simulink model "rigidBodyPD"  (Simulink 6.1)
settings: Solver=ode45  StartTime=0.0  StopTime=20.0  RelTol=1e-3
libraries: simulink x7
settings Model: LastModifiedBy=okawa
settings DebuggingCC: SolverPrmCheckMsg=warning

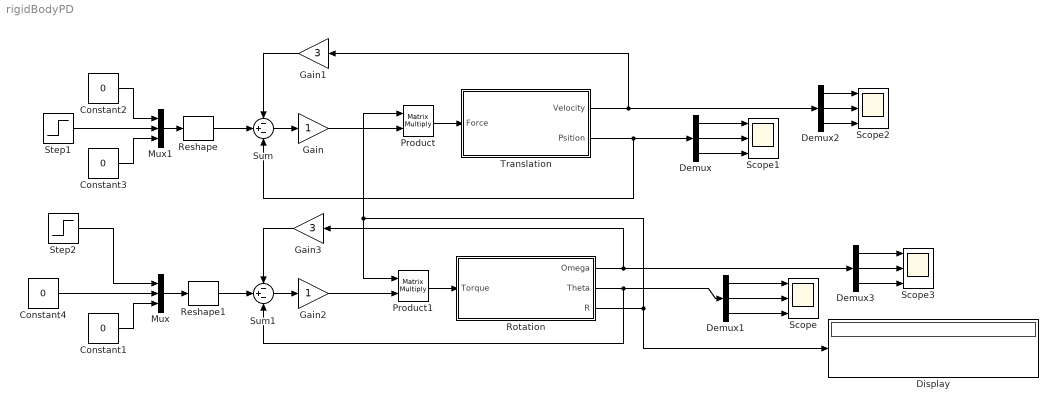
== system rigidBodyPD ==
  Constant{1..4} (4 alike) : Constant  Value=0
  Demux{,1..3} (4 alike) : Demux  Outputs=3
  Display : Display
  Gain : Gain
  Gain1 : Gain  Orientation=left  Gain=3
  Gain2 : Gain
  Gain3 : Gain  Orientation=left  Gain=3
  Mux : Mux  Inputs=3
  Mux1 : Mux  Inputs=3
  Product : Product  Multiplication=Matrix(*)  RndMeth=Zero
  Product1 : Product  Multiplication=Matrix(*)  RndMeth=Zero
  Reshape : simulink/Math Operations/Reshape  OutputDimensionality=Column vector  OutputDimensions=[1,1]
  Reshape1 : simulink/Math Operations/Reshape  OutputDimensionality=Column vector  OutputDimensions=[1,1]
  Rotation : Subsystem
  Scope{,1..3} (4 alike) : Scope  NumInputPorts=3
      Scope settings: YMin=-5~-5~-5  YMax=5~5~5
      Scope1 settings: YMin=-5~-5~-5  YMax=5~5~5
      Scope2 settings: YMin=-5~-5~-5  YMax=5~5~5  SaveName=ScopeData2
      Scope3 settings: YMin=-5~-5~-5  YMax=5~5~5  SaveName=ScopeData3
  Step1 : Step  SampleTime=0
  Step2 : Step  After=0.5  SampleTime=0
  Sum : Sum  Inputs=-+-
  Sum1 : Sum  Inputs=-+-
  Translation : Subsystem
  wires:
  Constant1/1 -> Mux/3
  Constant2/1 -> Mux1/1
  Step1/1 -> Mux1/2
  Constant3/1 -> Mux1/3
  Mux1/1 -> Reshape/1
  Product/1 -> Translation/1(Force)
  Demux1/1 -> Scope/1
  Demux1/2 -> Scope/2
  Demux1/3 -> Scope/3
  Mux/1 -> Reshape1/1
  Product1/1 -> Rotation/1(Torque)
  Translation/2(Psition) -> Demux/1, Sum/3
  Demux2/1 -> Scope2/1
  Demux2/2 -> Scope2/2
  Demux2/3 -> Scope2/3
  Translation/1(Velocity) -> Demux2/1, Gain1/1
  Demux/1 -> Scope1/1
  Demux/2 -> Scope1/2
  Demux/3 -> Scope1/3
  Demux3/1 -> Scope3/1
  Demux3/2 -> Scope3/2
  Demux3/3 -> Scope3/3
  Rotation/1(Omega) -> Demux3/1, Gain3/1
  Rotation/3(R) -> Product/1, Product1/1, Display/1
  Rotation/2(Theta) -> Demux1/1, Sum1/3
  Sum/1 -> Gain/1
  Gain/1 -> Product/2
  Reshape/1 -> Sum/2
  Gain1/1 -> Sum/1
  Reshape1/1 -> Sum1/2
  Sum1/1 -> Gain2/1
  Gain2/1 -> Product1/2
  Gain3/1 -> Sum1/1
  Step2/1 -> Mux/1
  Constant4/1 -> Mux/2

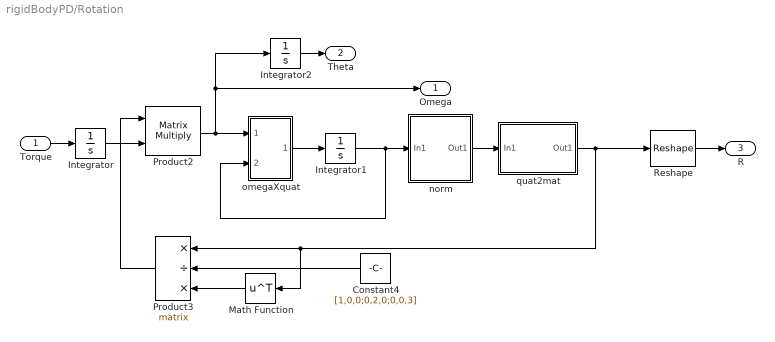
== system rigidBodyPD/Rotation ==
  Torque : Inport  Port=1  LatchInput=off
  Constant4 : Constant  Orientation=left  Value=[1,0,0;0,2,0;0,0,3]  VectorParams1D=off
  Integrator : Integrator
  Integrator1 : Integrator  InitialCondition=[1;0;0;0]
  Integrator2 : Integrator
  Math Function : Math  Orientation=left  Operator=transpose  SaturateOnIntegerOverflow=on
  Product2 : Product  Multiplication=Matrix(*)  RndMeth=Zero
  Product3 : Product  Orientation=left  Inputs=*/*  Multiplication=Matrix(*)  RndMeth=Zero
  Reshape : simulink/Math Operations/Reshape  OutputDimensionality=Customize  OutputDimensions=[3,3]
  norm : Subsystem
  "omegaXquat " : Subsystem
  quat2mat : Subsystem
  Omega : Outport
  Theta : Outport  Port=2
  R : Outport  Port=3
  wires:
  Integrator/1 -> Product2/2
  Product3/1 -> Product2/1
  Product2/1 -> "omegaXquat "/1(In1), Integrator2/1, Omega/1
  "omegaXquat "/1(Out1) -> Integrator1/1
  Integrator1/1 -> "omegaXquat "/2(In2), norm/1(In1)
  quat2mat/1(Out1) -> Product3/1, Math Function/1, Reshape/1
  Constant4/1 -> Product3/2
  Math Function/1 -> Product3/3
  norm/1(Out1) -> quat2mat/1(In1)
  Integrator2/1 -> Theta/1
  Torque/1 -> Integrator/1
  Reshape/1 -> R/1

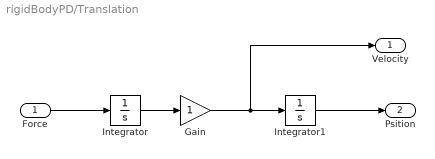
== system rigidBodyPD/Translation ==
  Force : Inport  Port=1  LatchInput=off
  Gain : Gain
  Integrator : Integrator
  Integrator1 : Integrator
  Velocity : Outport
  Psition : Outport  Port=2
  wires:
  Integrator/1 -> Gain/1
  Gain/1 -> Integrator1/1, Velocity/1
  Force/1 -> Integrator/1
  Integrator1/1 -> Psition/1

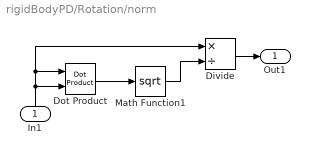
== system rigidBodyPD/Rotation/norm ==
  In1 : Inport  Orientation=up  Port=1  LatchInput=off
  Divide : Product  Inputs=*/  OutScaling=2^-10
  Dot Product : simulink/Math Operations/Dot Product  InputSameDT=on  OutDataType=sfix(16)  OutScaling=2^-10  DoSatur=off
  Math Function1 : Math  Operator=sqrt  SaturateOnIntegerOverflow=on
  Out1 : Outport
  wires:
  Dot Product/1 -> Math Function1/1
  Math Function1/1 -> Divide/2
  In1/1 -> Dot Product/2, Dot Product/1, Divide/1
  Divide/1 -> Out1/1

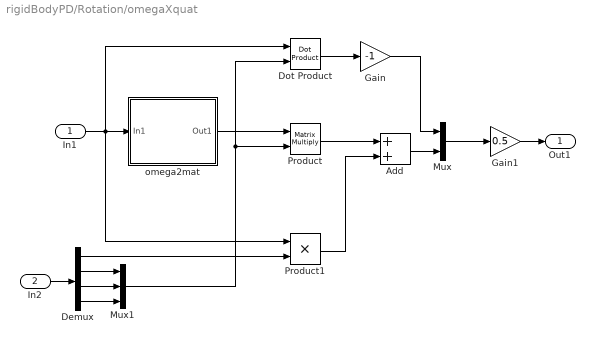
== system rigidBodyPD/Rotation/omegaXquat  ==
  In1 : Inport  Port=1  LatchInput=off
  In2 : Inport  Port=2  LatchInput=off
  Add : Sum  OutScaling=2^-10
  Demux : Demux
  Dot Product : simulink/Math Operations/Dot Product  InputSameDT=on  OutDataType=sfix(16)  OutScaling=2^-10  DoSatur=off
  Gain : Gain  Gain=-1
  Gain1 : Gain  Gain=0.5
  Mux : Mux  Inputs=2
  Mux1 : Mux  Inputs=3
  Product : Product  Multiplication=Matrix(*)  RndMeth=Zero
  Product1 : Product  RndMeth=Zero
  omega2mat : Subsystem
  Out1 : Outport
  wires:
  In1/1 -> Product1/1, Dot Product/1, omega2mat/1(In1)
  Dot Product/1 -> Gain/1
  omega2mat/1(Out1) -> Product/1
  Product/1 -> Add/1
  Product1/1 -> Add/2
  Gain/1 -> Mux/1
  Add/1 -> Mux/2
  Mux/1 -> Gain1/1
  Demux/2 -> Mux1/1
  Demux/3 -> Mux1/2
  Demux/4 -> Mux1/3
  Mux1/1 -> Dot Product/2, Product/2
  Demux/1 -> Product1/2
  Gain1/1 -> Out1/1
  In2/1 -> Demux/1

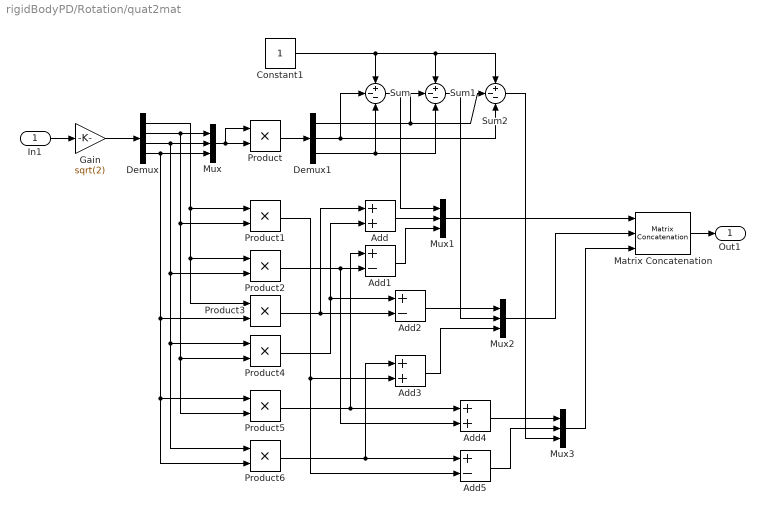
== system rigidBodyPD/Rotation/quat2mat ==
  In1 : Inport  Port=1  LatchInput=off
  Add : Sum  OutScaling=2^-10
  Add1 : Sum  Inputs=+-  OutScaling=2^-10
  Add2 : Sum  Inputs=+-  OutScaling=2^-10
  Add3 : Sum  OutScaling=2^-10
  Add4 : Sum  OutScaling=2^-10
  Add5 : Sum  Inputs=+-  OutScaling=2^-10
  Constant1 : Constant
  Demux : Demux
  Demux1 : Demux  Outputs=3
  Gain : Gain  Gain=sqrt(2)
  Matrix Concatenation : simulink/Math Operations/Matrix Concatenation  numInports=3  catMethod=Horizontal
  Mux{,1..3} (4 alike) : Mux  Inputs=3
  Product{,1..6} (7 alike) : Product  RndMeth=Zero
  Sum : Sum  Inputs=+--
  Sum1 : Sum  Inputs=+--
  Sum2 : Sum  Inputs=+--
  Out1 : Outport
  wires:
  Gain/1 -> Demux/1
  Demux/2 -> Mux/1, Product1/2, Product5/2, Product4/2
  Demux/3 -> Mux/2, Product6/1, Product4/1, Product2/2
  Demux/4 -> Mux/3, Product6/2, Product5/1, Product3/2
  Mux/1 -> Product/2, Product/1
  Product/1 -> Demux1/1
  Constant1/1 -> Sum/1, Sum2/1, Sum1/1
  Demux1/1 -> Sum2/2, Sum1/2
  Demux1/2 -> Sum2/3, Sum/2
  Demux1/3 -> Sum1/3, Sum/3
  Demux/1 -> Product1/1, Product3/1, Product2/1
  Mux1/1 -> Matrix Concatenation/1
  Mux3/1 -> Matrix Concatenation/3
  Mux2/1 -> Matrix Concatenation/2
  Add4/1 -> Mux3/1
  Add5/1 -> Mux3/2
  Sum2/1 -> Mux3/3
  Product6/1 -> Add5/1, Add3/1
  Product1/1 -> Add5/2, Add3/2
  Product5/1 -> Add4/1, Add1/1
  Add2/1 -> Mux2/1
  Sum1/1 -> Mux2/2
  Add3/1 -> Mux2/3
  Sum/1 -> Mux1/1
  Add/1 -> Mux1/2
  Add1/1 -> Mux1/3
  Product3/1 -> Add2/2, Add/1
  Product4/1 -> Add/2, Add2/1
  Product2/1 -> Add1/2, Add4/2
  In1/1 -> Gain/1
  Matrix Concatenation/1 -> Out1/1

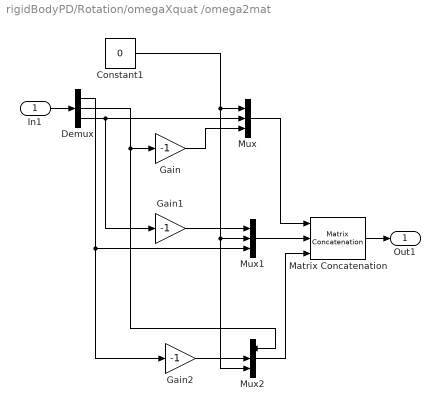
== system rigidBodyPD/Rotation/omegaXquat /omega2mat ==
  In1 : Inport  Port=1  LatchInput=off
  Constant1 : Constant  Value=0
  Demux : Demux  Outputs=3
  Gain : Gain  Gain=-1
  Gain1 : Gain  Gain=-1
  Gain2 : Gain  Gain=-1
  Matrix Concatenation : simulink/Math Operations/Matrix Concatenation  numInports=3  catMethod=Horizontal
  Mux : Mux  Inputs=3
  Mux1 : Mux  Inputs=3
  Mux2 : Mux  Inputs=3
  Out1 : Outport
  wires:
  Constant1/1 -> Mux/1, Mux1/2, Mux2/3
  Demux/2 -> Gain/1, Mux2/1
  Gain/1 -> Mux/3
  Demux/3 -> Mux/2, Gain1/1
  Gain1/1 -> Mux1/1
  Demux/1 -> Mux1/3, Gain2/1
  Gain2/1 -> Mux2/2
  Mux/1 -> Matrix Concatenation/1
  Mux1/1 -> Matrix Concatenation/2
  Mux2/1 -> Matrix Concatenation/3
  In1/1 -> Demux/1
  Matrix Concatenation/1 -> Out1/1
